simulink model "UZ_EnDat_be4_adding_bidirectional_clk_shift"  (R2024a)
settings: Solver=FixedStepDiscrete  StartTime=0  StopTime=0.02  FixedStep=1.0E-8  RelTol=1e-3
model workspace (MAT data in the model file):
  Select = 0
libraries: hdlsllib x776, simulink x28, simulink_extras x3
(part 4 of 9)

== system UZ_EnDat_be4_adding_bidirectional_clk_shift/UZ_ENDAT/ManualSerializeWrap/ManualSerializer ==
  CLK : Inport
  SLOWCLCK : Inport  Port=2
  DATA : Inport  Port=3
  reset : Inport  Port=4
  Constant3 : Constant  Value=0  OutDataTypeStr=boolean  SampleTime=-1
  Delay1 : Delay  DelayLength=1
  Multiport Switch : MultiPortSwitch  Inputs=6  DataPortForDefault=Additional data port  DiagnosticForDefault=None  SaturateOnIntegerOverflow=off  InputSameDT=off
  Terminator{1..10} (10 alike) : Terminator
  WORDTOBOOL : Subsystem  TreatAsAtomicUnit=on
  ramwatcher : Subsystem  TreatAsAtomicUnit=on
      settings: LibrarySourceBlock=|
      | hdlsllib/Ports &
      | Subsystems/Triggered
      | Subsystem
  valin : Outport
  wires:
  SLOWCLCK/1 -> ramwatcher/Trigger
  DATA/1 -> WORDTOBOOL/1(DATAIN)
  Multiport Switch/1 -> valin/1
  CLK/1 -> WORDTOBOOL/Trigger
  Delay1/1 -> ramwatcher/1(In1)
  Constant3/1 -> Multiport Switch/8
  reset/1 -> ramwatcher/2(reset)
  WORDTOBOOL/1(DATAOUT0) -> Multiport Switch/7
  WORDTOBOOL/2(DATAOUT1) -> Multiport Switch/6
  WORDTOBOOL/3(DATAOUT2) -> Multiport Switch/5
  WORDTOBOOL/4(DATAOUT3) -> Multiport Switch/4
  WORDTOBOOL/5(DATAOUT4) -> Multiport Switch/3
  WORDTOBOOL/6(DATAOUT5) -> Multiport Switch/2
  WORDTOBOOL/9(DATAOUT8) -> Terminator2/1
  WORDTOBOOL/10(DATAOUT9) -> Terminator3/1
  WORDTOBOOL/11(DATAOUT10) -> Terminator4/1
  WORDTOBOOL/12(DATAOUT11) -> Terminator5/1
  WORDTOBOOL/13(DATAOUT12) -> Terminator6/1
  WORDTOBOOL/14(DATAOUT13) -> Terminator7/1
  WORDTOBOOL/15(DATAOUT14) -> Terminator8/1
  WORDTOBOOL/16(DATAOUT15) -> Terminator9/1
  WORDTOBOOL/7(DATAOUT6) -> Terminator1/1
  WORDTOBOOL/8(DATAOUT7) -> Terminator10/1
  ramwatcher/1(SEL) -> Multiport Switch/1, Delay1/1

== system UZ_EnDat_be4_adding_bidirectional_clk_shift/UZ_ENDAT/RESPONSESLICER3X/19BITSLICER ==
  DATA : Inport
  DATA1 : Inport  Port=2
  DATA2 : Inport  Port=3
  Enable : EnablePort
  Terminator : Terminator
  Terminator1 : Terminator
  responseslicer : Subsystem
      settings: LibrarySourceBlock=|
      | hdlsllib/Ports &
      | Subsystems/Subsystem
  responseslicer1 : Subsystem
      settings: LibrarySourceBlock=|
      | hdlsllib/Ports &
      | Subsystems/Subsystem
  responseslicer2 : Subsystem
      settings: LibrarySourceBlock=|
      | hdlsllib/Ports &
      | Subsystems/Subsystem
  CRC : Outport  InitialOutput=0
  payload : Outport  Port=2  InitialOutput=0
  CRC1 : Outport  Port=3  InitialOutput=0
  payload1 : Outport  Port=4  InitialOutput=0
  CRC2 : Outport  Port=5  InitialOutput=0
  payload2 : Outport  Port=6  InitialOutput=0
  sensorerror : Outport  Port=7  InitialOutput=0
  wires:
  DATA1/1 -> responseslicer1/1(DATA)
  DATA/1 -> responseslicer/1(DATA)
  responseslicer/2(payload) -> payload/1
  responseslicer1/2(payload) -> payload1/1
  responseslicer2/2(payload) -> payload2/1
  responseslicer/1(CRC) -> CRC/1
  DATA2/1 -> responseslicer2/1(DATA)
  responseslicer1/1(CRC) -> CRC1/1
  responseslicer2/1(CRC) -> CRC2/1
  responseslicer/3(error) -> sensorerror/1
  responseslicer1/3(error) -> Terminator/1
  responseslicer2/3(error) -> Terminator1/1

== system UZ_EnDat_be4_adding_bidirectional_clk_shift/UZ_ENDAT/RESPONSESLICER3X/21BITSLICER ==
  DATA : Inport
  DATA1 : Inport  Port=2
  DATA2 : Inport  Port=3
  Enable : EnablePort
  Terminator : Terminator
  Terminator1 : Terminator
  responseslicer : Subsystem
      settings: LibrarySourceBlock=|
      | hdlsllib/Ports &
      | Subsystems/Subsystem
  responseslicer3 : Subsystem
      settings: LibrarySourceBlock=|
      | hdlsllib/Ports &
      | Subsystems/Subsystem
  responseslicer4 : Subsystem
      settings: LibrarySourceBlock=|
      | hdlsllib/Ports &
      | Subsystems/Subsystem
  CRC : Outport  InitialOutput=0
  payload : Outport  Port=2  InitialOutput=0
  CRC1 : Outport  Port=3  InitialOutput=0
  payload1 : Outport  Port=4  InitialOutput=0
  CRC2 : Outport  Port=5  InitialOutput=0
  payload2 : Outport  Port=6  InitialOutput=0
  sensorerror : Outport  Port=7  InitialOutput=0
  wires:
  DATA1/1 -> responseslicer4/1(DATA)
  DATA/1 -> responseslicer/1(DATA)
  responseslicer/2(payload) -> payload/1
  responseslicer4/2(payload) -> payload1/1
  responseslicer3/2(payload) -> payload2/1
  responseslicer/1(CRC) -> CRC/1
  DATA2/1 -> responseslicer3/1(DATA)
  responseslicer4/1(CRC) -> CRC1/1
  responseslicer3/1(CRC) -> CRC2/1
  responseslicer/3(error) -> sensorerror/1
  responseslicer4/3(error) -> Terminator/1
  responseslicer3/3(error) -> Terminator1/1

== system UZ_EnDat_be4_adding_bidirectional_clk_shift/UZ_ENDAT/RESPONSESLICER3X/23BITSLICER ==
  DATA : Inport
  DATA1 : Inport  Port=2
  DATA2 : Inport  Port=3
  Enable : EnablePort
  Terminator : Terminator
  Terminator1 : Terminator
  responseslicer : Subsystem
      settings: LibrarySourceBlock=|
      | hdlsllib/Ports &
      | Subsystems/Subsystem
  responseslicer1 : Subsystem
      settings: LibrarySourceBlock=|
      | hdlsllib/Ports &
      | Subsystems/Subsystem
  responseslicer2 : Subsystem
      settings: LibrarySourceBlock=|
      | hdlsllib/Ports &
      | Subsystems/Subsystem
  CRC : Outport  InitialOutput=0
  payload : Outport  Port=2  InitialOutput=0
  CRC1 : Outport  Port=3  InitialOutput=0
  payload1 : Outport  Port=4  InitialOutput=0
  CRC2 : Outport  Port=5  InitialOutput=0
  payload2 : Outport  Port=6  InitialOutput=0
  sensorerror : Outport  Port=7  InitialOutput=0
  wires:
  DATA1/1 -> responseslicer1/1(DATA)
  DATA/1 -> responseslicer/1(DATA)
  responseslicer/2(payload) -> payload/1
  responseslicer1/2(payload) -> payload1/1
  responseslicer2/2(payload) -> payload2/1
  responseslicer/1(CRC) -> CRC/1
  DATA2/1 -> responseslicer2/1(DATA)
  responseslicer1/1(CRC) -> CRC1/1
  responseslicer2/1(CRC) -> CRC2/1
  responseslicer/3(error) -> sensorerror/1
  responseslicer1/3(error) -> Terminator/1
  responseslicer2/3(error) -> Terminator1/1

== system UZ_EnDat_be4_adding_bidirectional_clk_shift/UZ_ENDAT/RESPONSESLICER3X/25BITSLICER ==
  DATA : Inport
  DATA1 : Inport  Port=2
  DATA2 : Inport  Port=3
  Enable : EnablePort
  Terminator : Terminator
  Terminator1 : Terminator
  responseslicer : Subsystem
      settings: LibrarySourceBlock=|
      | hdlsllib/Ports &
      | Subsystems/Subsystem
  responseslicer1 : Subsystem
      settings: LibrarySourceBlock=|
      | hdlsllib/Ports &
      | Subsystems/Subsystem
  responseslicer2 : Subsystem
      settings: LibrarySourceBlock=|
      | hdlsllib/Ports &
      | Subsystems/Subsystem
  CRC : Outport  InitialOutput=0
  payload : Outport  Port=2  InitialOutput=0
  CRC1 : Outport  Port=3  InitialOutput=0
  payload1 : Outport  Port=4  InitialOutput=0
  CRC2 : Outport  Port=5  InitialOutput=0
  payload2 : Outport  Port=6  InitialOutput=0
  sensorerror : Outport  Port=7  InitialOutput=0
  wires:
  DATA1/1 -> responseslicer1/1(DATA)
  DATA/1 -> responseslicer/1(DATA)
  responseslicer/2(payload) -> payload/1
  responseslicer1/2(payload) -> payload1/1
  responseslicer2/2(payload) -> payload2/1
  responseslicer/1(CRC) -> CRC/1
  DATA2/1 -> responseslicer2/1(DATA)
  responseslicer1/1(CRC) -> CRC1/1
  responseslicer2/1(CRC) -> CRC2/1
  responseslicer/3(error) -> sensorerror/1
  responseslicer1/3(error) -> Terminator/1
  responseslicer2/3(error) -> Terminator1/1

== system UZ_EnDat_be4_adding_bidirectional_clk_shift/UZ_ENDAT/RESPONSESLICER3X/27BITSLICER ==
  DATA : Inport
  DATA1 : Inport  Port=2
  DATA2 : Inport  Port=3
  Enable : EnablePort
  Terminator : Terminator
  Terminator1 : Terminator
  responseslicer : Subsystem
      settings: LibrarySourceBlock=|
      | hdlsllib/Ports &
      | Subsystems/Subsystem
  responseslicer1 : Subsystem
      settings: LibrarySourceBlock=|
      | hdlsllib/Ports &
      | Subsystems/Subsystem
  responseslicer2 : Subsystem
      settings: LibrarySourceBlock=|
      | hdlsllib/Ports &
      | Subsystems/Subsystem
  CRC : Outport  InitialOutput=0
  payload : Outport  Port=2  InitialOutput=0
  CRC1 : Outport  Port=3  InitialOutput=0
  payload1 : Outport  Port=4  InitialOutput=0
  CRC2 : Outport  Port=5  InitialOutput=0
  payload2 : Outport  Port=6  InitialOutput=0
  sensorerror : Outport  Port=7  InitialOutput=0
  wires:
  DATA1/1 -> responseslicer1/1(DATA)
  DATA/1 -> responseslicer/1(DATA)
  responseslicer/2(payload) -> payload/1
  responseslicer1/2(payload) -> payload1/1
  responseslicer2/2(payload) -> payload2/1
  responseslicer/1(CRC) -> CRC/1
  DATA2/1 -> responseslicer2/1(DATA)
  responseslicer1/1(CRC) -> CRC1/1
  responseslicer2/1(CRC) -> CRC2/1
  responseslicer/3(error) -> sensorerror/1
  responseslicer1/3(error) -> Terminator/1
  responseslicer2/3(error) -> Terminator1/1

== system UZ_EnDat_be4_adding_bidirectional_clk_shift/UZ_ENDAT/timingprovider/Subsystem1 ==
  Trigger : TriggerPort  VariantControl=(inherit)  PortDimensions=1
  HDL Counter : hdlsllib/Sources/HDL Counter  CountType=Count limited  CountInit=0  CountStep=1  CountMax=3  CountFromType=Initial value  CountFrom=0  CountResetPort=off  CountLoadPort=off  CountEnbPort=off  CountDirPort=off  CountHitOutputPort=on  CountDataType=Unsigned  CountWordLen=2  CountFracLen=0  CountSampTime=-1
  valin1 : Outport  InitialOutput=0
  valin2 : Outport  Port=2  InitialOutput=0
  wires:
  HDL Counter/1 -> valin1/1
  HDL Counter/2 -> valin2/1

== system UZ_EnDat_be4_adding_bidirectional_clk_shift/UZ_ENDAT/timingprovider/Subsystem2 ==
  elapsed : Inport
  clkcnt : Inport  Port=2
  Compare To Constant1 : hdlsllib/Logic and Bit Operations/Compare To Constant  relop===  const=3  OutDataTypeStr=boolean
  Delay1 : Delay  DelayLength=1
  Detect Increase : simulink/Logic and Bit Operations/Detect Increase  vinit=0  OutDataTypeStr=boolean
      settings: LibrarySourceBlock=|
      | hdlsllib/Logic and Bit
      | Operations/Detect
      | Increase
  Gain : Gain  Gain=10  ParamMin=10  ParamMax=10  ParamDataTypeStr=uint8  OutDataTypeStr=uint32  RndMeth=Simplest
  Switch : Switch  Criteria=u2 > Threshold  SaturateOnIntegerOverflow=off  InputSameDT=off
  ns elapsed : Outport
  wires:
  Detect Increase/1 -> Switch/2
  clkcnt/1 -> Switch/1
  Switch/1 -> Gain/1, Delay1/1
  Delay1/1 -> Switch/3
  elapsed/1 -> Compare To Constant1/1
  Gain/1 -> ns elapsed/1  "ns elapsed"
  Compare To Constant1/1 -> Detect Increase/1

== system UZ_EnDat_be4_adding_bidirectional_clk_shift/UZ_ENDAT/timingprovider/Subsystem3 ==
  elapsed : Inport
  clkcnt : Inport  Port=2
  Compare To Constant1 : hdlsllib/Logic and Bit Operations/Compare To Constant  relop===  const=3  OutDataTypeStr=boolean
  Constant : Constant  Value=10  OutDataTypeStr=uint8  SampleTime=-1
  Delay1 : Delay  DelayLength=1
  Detect Increase : simulink/Logic and Bit Operations/Detect Increase  vinit=0  OutDataTypeStr=boolean
      settings: LibrarySourceBlock=|
      | hdlsllib/Logic and Bit
      | Operations/Detect
      | Increase
  Switch : Switch  Criteria=u2 > Threshold  SaturateOnIntegerOverflow=off  InputSameDT=off
  nsproduct : Product  OutDataTypeStr=uint32  RndMeth=Simplest
  ns elapsed : Outport
  wires:
  Detect Increase/1 -> Switch/2
  clkcnt/1 -> Switch/1
  Switch/1 -> nsproduct/2, Delay1/1
  Delay1/1 -> Switch/3
  elapsed/1 -> Compare To Constant1/1
  nsproduct/1 -> ns elapsed/1  "ns elapsed"
  Constant/1 -> nsproduct/1
  Compare To Constant1/1 -> Detect Increase/1

== system UZ_EnDat_be4_adding_bidirectional_clk_shift/UZ_ENDAT/timingprovider/Subsystem4 ==
  reset : Inport
  Trigger : TriggerPort  TriggerType=either  VariantControl=(inherit)  PortDimensions=1
  Delay : Delay  Commented=through  DelayLength=1
  HDL Counter : hdlsllib/Sources/HDL Counter  CountType=Count limited  CountInit=0  CountStep=1  CountMax=65535  CountFromType=Initial value  CountFrom=0  CountResetPort=on  CountLoadPort=off  CountEnbPort=off  CountDirPort=off  CountHitOutputPort=off  CountDataType=Unsigned  CountWordLen=16  CountFracLen=0  CountSampTime=1
  Scope : Scope
  valin1 : Outport  InitialOutput=0
  wires:
  reset/1 -> Delay/1
  HDL Counter/1 -> valin1/1, Scope/1
  Delay/1 -> HDL Counter/1

== system UZ_EnDat_be4_adding_bidirectional_clk_shift/UZ_ENDAT/timingprovider/Subsystem5 ==
  elapsed : Inport
  clkcnt : Inport  Port=2
  Compare To Constant1 : hdlsllib/Logic and Bit Operations/Compare To Constant  relop===  const=2  OutDataTypeStr=boolean
  Delay1 : Delay  DelayLength=1
  Detect Increase : simulink/Logic and Bit Operations/Detect Increase  vinit=0  OutDataTypeStr=boolean
      settings: LibrarySourceBlock=|
      | hdlsllib/Logic and Bit
      | Operations/Detect
      | Increase
  Gain : Gain  Gain=10  ParamMin=10  ParamMax=10  ParamDataTypeStr=uint8  OutDataTypeStr=uint32  RndMeth=Simplest
  Switch : Switch  Criteria=u2 > Threshold  SaturateOnIntegerOverflow=off  InputSameDT=off
  ns elapsed : Outport
  wires:
  Detect Increase/1 -> Switch/2
  clkcnt/1 -> Switch/1
  Switch/1 -> Gain/1, Delay1/1
  Delay1/1 -> Switch/3
  elapsed/1 -> Compare To Constant1/1
  Gain/1 -> ns elapsed/1  "ns elapsed"
  Compare To Constant1/1 -> Detect Increase/1

== system UZ_EnDat_be4_adding_bidirectional_clk_shift/UZ_ENDAT/timingprovider/Subsystem6 ==
  elapsed : Inport
  clkcnt : Inport  Port=2
  Compare To Constant1 : hdlsllib/Logic and Bit Operations/Compare To Constant  relop===  const=3  OutDataTypeStr=boolean
  Constant : Constant  Value=10  OutDataTypeStr=uint8  SampleTime=-1
  Delay1 : Delay  DelayLength=1
  Detect Increase : simulink/Logic and Bit Operations/Detect Increase  vinit=0  OutDataTypeStr=boolean
      settings: LibrarySourceBlock=|
      | hdlsllib/Logic and Bit
      | Operations/Detect
      | Increase
  Switch : Switch  Criteria=u2 > Threshold  SaturateOnIntegerOverflow=off  InputSameDT=off
  nsproduct : Product  OutDataTypeStr=uint32  RndMeth=Simplest
  ns elapsed : Outport
  wires:
  Detect Increase/1 -> Switch/2
  clkcnt/1 -> Switch/1
  Switch/1 -> nsproduct/2, Delay1/1
  Delay1/1 -> Switch/3
  elapsed/1 -> Compare To Constant1/1
  nsproduct/1 -> ns elapsed/1  "ns elapsed"
  Constant/1 -> nsproduct/1
  Compare To Constant1/1 -> Detect Increase/1

== system UZ_EnDat_be4_adding_bidirectional_clk_shift/UZ_ENDAT/timingprovider/Subsystem7 ==
  elapsed : Inport
  clkcnt : Inport  Port=2
  Compare To Constant1 : hdlsllib/Logic and Bit Operations/Compare To Constant  relop===  const=2  OutDataTypeStr=boolean
  Constant : Constant  Value=10  OutDataTypeStr=uint8  SampleTime=-1
  Delay1 : Delay  DelayLength=1
  Detect Increase : simulink/Logic and Bit Operations/Detect Increase  vinit=0  OutDataTypeStr=boolean
      settings: LibrarySourceBlock=|
      | hdlsllib/Logic and Bit
      | Operations/Detect
      | Increase
  Switch : Switch  Criteria=u2 > Threshold  SaturateOnIntegerOverflow=off  InputSameDT=off
  nsproduct : Product  OutDataTypeStr=uint32  RndMeth=Simplest
  ns elapsed : Outport
  wires:
  Detect Increase/1 -> Switch/2
  clkcnt/1 -> Switch/1
  Switch/1 -> nsproduct/2, Delay1/1
  Delay1/1 -> Switch/3
  elapsed/1 -> Compare To Constant1/1
  nsproduct/1 -> ns elapsed/1  "ns elapsed"
  Constant/1 -> nsproduct/1
  Compare To Constant1/1 -> Detect Increase/1

== system UZ_EnDat_be4_adding_bidirectional_clk_shift/UZ_ENDAT/timingprovideralternative/Subsystem1 ==
  Trigger : TriggerPort  VariantControl=(inherit)  PortDimensions=1
  HDL Counter : hdlsllib/Sources/HDL Counter  CountType=Count limited  CountInit=0  CountStep=1  CountMax=3  CountFromType=Initial value  CountFrom=0  CountResetPort=off  CountLoadPort=off  CountEnbPort=off  CountDirPort=off  CountHitOutputPort=on  CountDataType=Unsigned  CountWordLen=2  CountFracLen=0  CountSampTime=-1
  valin1 : Outport  InitialOutput=0
  valin2 : Outport  Port=2  InitialOutput=0
  wires:
  HDL Counter/1 -> valin1/1
  HDL Counter/2 -> valin2/1

== system UZ_EnDat_be4_adding_bidirectional_clk_shift/UZ_ENDAT/timingprovideralternative/Subsystem2 ==
  elapsed : Inport
  clkcnt : Inport  Port=2
  Compare To Constant1 : hdlsllib/Logic and Bit Operations/Compare To Constant  relop===  const=3  OutDataTypeStr=boolean
  Constant : Constant  Value=10  OutDataTypeStr=uint32  SampleTime=-1
  Delay1 : Delay  DelayLength=1
  Detect Increase : simulink/Logic and Bit Operations/Detect Increase  vinit=0  OutDataTypeStr=boolean
      settings: LibrarySourceBlock=|
      | hdlsllib/Logic and Bit
      | Operations/Detect
      | Increase
  Switch : Switch  Criteria=u2 > Threshold  SaturateOnIntegerOverflow=off  InputSameDT=off
  nsproduct : Product  OutDataTypeStr=uint32  RndMeth=Simplest  SaturateOnIntegerOverflow=on
  ns elapsed : Outport
  wires:
  Detect Increase/1 -> Switch/2
  clkcnt/1 -> Switch/1
  Switch/1 -> nsproduct/2, Delay1/1
  Delay1/1 -> Switch/3
  elapsed/1 -> Compare To Constant1/1
  nsproduct/1 -> ns elapsed/1  "ns elapsed"
  Constant/1 -> nsproduct/1
  Compare To Constant1/1 -> Detect Increase/1

== system UZ_EnDat_be4_adding_bidirectional_clk_shift/UZ_ENDAT/timingprovideralternative/Subsystem3 ==
  elapsed : Inport
  clkcnt : Inport  Port=2
  Compare To Constant1 : hdlsllib/Logic and Bit Operations/Compare To Constant  relop===  const=2  OutDataTypeStr=boolean
  Constant : Constant  Value=10  OutDataTypeStr=uint32  SampleTime=-1
  Delay1 : Delay  DelayLength=1
  Detect Increase : simulink/Logic and Bit Operations/Detect Increase  vinit=0  OutDataTypeStr=boolean
      settings: LibrarySourceBlock=|
      | hdlsllib/Logic and Bit
      | Operations/Detect
      | Increase
  Switch : Switch  Criteria=u2 > Threshold  SaturateOnIntegerOverflow=off  InputSameDT=off
  nsproduct : Product  OutDataTypeStr=uint32  RndMeth=Simplest  SaturateOnIntegerOverflow=on
  ns elapsed : Outport
  wires:
  Detect Increase/1 -> Switch/2
  clkcnt/1 -> Switch/1
  Switch/1 -> nsproduct/2, Delay1/1
  Delay1/1 -> Switch/3
  elapsed/1 -> Compare To Constant1/1
  nsproduct/1 -> ns elapsed/1  "ns elapsed"
  Constant/1 -> nsproduct/1
  Compare To Constant1/1 -> Detect Increase/1

== system UZ_EnDat_be4_adding_bidirectional_clk_shift/UZ_ENDAT/timingprovideralternative/Subsystem4 ==
  reset : Inport
  Delay : Delay  Commented=through  DelayLength=1
  HDL Counter : hdlsllib/Sources/HDL Counter  CountType=Count limited  CountInit=0  CountStep=1  CountMax=214748364  CountFromType=Initial value  CountFrom=0  CountResetPort=on  CountLoadPort=off  CountEnbPort=off  CountDirPort=off  CountHitOutputPort=off  CountDataType=Unsigned  CountWordLen=32  CountFracLen=0  CountSampTime=1
  Scope : Scope
  valin1 : Outport  InitialOutput=0
  wires:
  reset/1 -> Delay/1
  HDL Counter/1 -> valin1/1, Scope/1
  Delay/1 -> HDL Counter/1

== system UZ_EnDat_be4_adding_bidirectional_clk_shift/UZ_ENDAT/timingprovideralternative/timingproviderold ==
  wrok : Inport  OutDataTypeStr=boolean
  clk : Inport  Port=2  OutDataTypeStr=boolean
  Compare To Constant1 : hdlsllib/Logic and Bit Operations/Compare To Constant  relop===  const=0  OutDataTypeStr=boolean
  Constant3 : Constant  Commented=on  Value=0x7FFFF0  OutDataTypeStr=uint32  SampleTime=-1
  Constant4 : Constant  Commented=on  Value=0x7FFFFF  OutDataTypeStr=uint32  SampleTime=-1
  Logical Operator : Logic  Operator=OR  AllPortsSameDT=off  OutDataTypeStr=boolean
  Subsystem1 : Subsystem
  Subsystem2 : Subsystem
  Subsystem3 : Subsystem
  Subsystem4 : Subsystem
  timeelapsed2cycl : Outport  OutDataTypeStr=uint32
  timeelapsed1cycl : Outport  Port=2  OutDataTypeStr=uint32
  wires:
  wrok/1 -> Subsystem1/Trigger
  Subsystem2/1(ns elapsed) -> timeelapsed2cycl/1
  Subsystem3/1(ns elapsed) -> timeelapsed1cycl/1
  Subsystem1/1(valin1) -> Compare To Constant1/1, Subsystem3/1(elapsed), Subsystem2/1(elapsed)
  Logical Operator/1 -> Subsystem4/1(reset)
  Compare To Constant1/1 -> Logical Operator/2
  clk/1 -> Subsystem4/Trigger
  Subsystem4/1(valin1) -> Subsystem2/2(clkcnt), Subsystem3/2(clkcnt)
  Subsystem1/2(valin2) -> Logical Operator/1

== system UZ_EnDat_be4_adding_bidirectional_clk_shift/UZ_ENDAT/timingproviderold1/Subsystem1 ==
  Trigger : TriggerPort  VariantControl=(inherit)  PortDimensions=1
  HDL Counter : hdlsllib/Sources/HDL Counter  CountType=Count limited  CountInit=0  CountStep=1  CountMax=3  CountFromType=Initial value  CountFrom=0  CountResetPort=off  CountLoadPort=off  CountEnbPort=off  CountDirPort=off  CountHitOutputPort=on  CountDataType=Unsigned  CountWordLen=2  CountFracLen=0  CountSampTime=-1
  valin1 : Outport  InitialOutput=0
  valin2 : Outport  Port=2  InitialOutput=0
  wires:
  HDL Counter/1 -> valin1/1
  HDL Counter/2 -> valin2/1

== system UZ_EnDat_be4_adding_bidirectional_clk_shift/UZ_ENDAT/timingproviderold1/Subsystem2 ==
  elapsed : Inport
  clkcnt : Inport  Port=2
  Compare To Constant1 : hdlsllib/Logic and Bit Operations/Compare To Constant  relop===  const=3  OutDataTypeStr=boolean
  Constant : Constant  Value=20  OutDataTypeStr=uint32  SampleTime=-1
  Delay1 : Delay  DelayLength=1
  Detect Increase : simulink/Logic and Bit Operations/Detect Increase  vinit=0  OutDataTypeStr=boolean
      settings: LibrarySourceBlock=|
      | hdlsllib/Logic and Bit
      | Operations/Detect
      | Increase
  Switch : Switch  Criteria=u2 > Threshold  SaturateOnIntegerOverflow=off  InputSameDT=off
  nsproduct : Product  OutDataTypeStr=uint32  RndMeth=Simplest  SaturateOnIntegerOverflow=on
  ns elapsed : Outport
  wires:
  Detect Increase/1 -> Switch/2
  clkcnt/1 -> Switch/1
  Switch/1 -> nsproduct/2, Delay1/1
  Delay1/1 -> Switch/3
  elapsed/1 -> Compare To Constant1/1
  nsproduct/1 -> ns elapsed/1  "ns elapsed"
  Constant/1 -> nsproduct/1
  Compare To Constant1/1 -> Detect Increase/1

== system UZ_EnDat_be4_adding_bidirectional_clk_shift/UZ_ENDAT/timingproviderold1/Subsystem3 ==
  elapsed : Inport
  clkcnt : Inport  Port=2
  Compare To Constant1 : hdlsllib/Logic and Bit Operations/Compare To Constant  relop===  const=2  OutDataTypeStr=boolean
  Constant : Constant  Value=20  OutDataTypeStr=uint32  SampleTime=-1
  Delay1 : Delay  DelayLength=1
  Detect Increase : simulink/Logic and Bit Operations/Detect Increase  vinit=0  OutDataTypeStr=boolean
      settings: LibrarySourceBlock=|
      | hdlsllib/Logic and Bit
      | Operations/Detect
      | Increase
  Switch : Switch  Criteria=u2 > Threshold  SaturateOnIntegerOverflow=off  InputSameDT=off
  nsproduct : Product  OutDataTypeStr=uint32  RndMeth=Simplest  SaturateOnIntegerOverflow=on
  ns elapsed : Outport
  wires:
  Detect Increase/1 -> Switch/2
  clkcnt/1 -> Switch/1
  Switch/1 -> nsproduct/2, Delay1/1
  Delay1/1 -> Switch/3
  elapsed/1 -> Compare To Constant1/1
  nsproduct/1 -> ns elapsed/1  "ns elapsed"
  Constant/1 -> nsproduct/1
  Compare To Constant1/1 -> Detect Increase/1

== system UZ_EnDat_be4_adding_bidirectional_clk_shift/UZ_ENDAT/timingproviderold1/Subsystem4 ==
  reset : Inport
  Trigger : TriggerPort  VariantControl=(inherit)  PortDimensions=1
  Delay : Delay  Commented=through  DelayLength=1
  HDL Counter : hdlsllib/Sources/HDL Counter  CountType=Count limited  CountInit=0  CountStep=1  CountMax=214748364  CountFromType=Initial value  CountFrom=0  CountResetPort=on  CountLoadPort=off  CountEnbPort=off  CountDirPort=off  CountHitOutputPort=off  CountDataType=Unsigned  CountWordLen=32  CountFracLen=0  CountSampTime=1
  Scope : Scope
  valin1 : Outport  InitialOutput=0
  wires:
  reset/1 -> Delay/1
  HDL Counter/1 -> valin1/1, Scope/1
  Delay/1 -> HDL Counter/1

== system UZ_EnDat_be4_adding_bidirectional_clk_shift/UZ_ENDAT_ABZ_ADDON/ManualSerialize1/FF1 ==
  SET : Inport
  RST : Inport  Port=2
  S-R Flip-Flop : simulink_extras/Flip Flops/S-R Flip-Flop  initial_condition=0
  OQ : Outport
  NOQ : Outport  Port=2
  wires:
  SET/1 -> S-R Flip-Flop/1
  RST/1 -> S-R Flip-Flop/2
  S-R Flip-Flop/1 -> OQ/1
  S-R Flip-Flop/2 -> NOQ/1

== system UZ_EnDat_be4_adding_bidirectional_clk_shift/UZ_ENDAT_ABZ_ADDON/ManualSerialize1/SetZero64modified ==
  valin : Inport
  setzero : Inport  Port=2  OutDataTypeStr=boolean
  Trigger : TriggerPort  TriggerType=either  VariantControl=(inherit)
  Constant2 : Constant  Value=0  OutDataTypeStr=uint64  SampleTime=-1
  Index Vector1 : MultiPortSwitch  DataPortOrder=Zero-based contiguous  Inputs=2  zeroidx=on  OutDataTypeStr=uint64  SaturateOnIntegerOverflow=off  InputSameDT=off
  valueout : Outport  InitialOutput=1  VectorParamsAs1DForOutWhenUnconnected=off
  wires:
  valin/1 -> Index Vector1/2
  Index Vector1/1 -> valueout/1
  Constant2/1 -> Index Vector1/3
  setzero/1 -> Index Vector1/1

== system UZ_EnDat_be4_adding_bidirectional_clk_shift/UZ_ENDAT_ABZ_ADDON/ManualSerialize1/Storage1 ==
  Data : Inport
  Write : Inport  Port=2  OutDataTypeStr=boolean
  Compare To Zero : hdlsllib/Logic and Bit Operations/Compare To Zero  relop===  OutDataTypeStr=boolean
  Delay2 : Delay  DelayLength=1
  Logical Operator1 : Logic  AllPortsSameDT=off  OutDataTypeStr=boolean
  Logical Operator2 : Logic  Operator=NOT  AllPortsSameDT=off  OutDataTypeStr=boolean
  Single Port RAM System : hdlsllib/HDL RAMs/Single Port RAM System  Commented=on  RAMType=Single port  AsyncRead=off  WriteOutputValue=Old data  RAMInitialValue=0  allowBusInputs=off  WritesHaveOutput=on  NumReads=0  NumWrites=1  SimulateUsing=Code generation
  Switch : Switch  Criteria=u2 > Threshold  SaturateOnIntegerOverflow=off  InputSameDT=off
  prolonger : Subsystem  Commented=through
  out : Outport
  wrok : Outport  Port=2  OutDataTypeStr=boolean
  wires:
  Switch/1 -> Delay2/1
  Compare To Zero/1 -> Logical Operator2/1
  Logical Operator2/1 -> Logical Operator1/2
  prolonger/1(out) -> wrok/1
  Data/1 -> Compare To Zero/1, Switch/1
  Delay2/1 -> out/1, Switch/3
  Logical Operator1/1 -> prolonger/1(in), Switch/2
  Write/1 -> Logical Operator1/1

== system UZ_EnDat_be4_adding_bidirectional_clk_shift/UZ_ENDAT_ABZ_ADDON/ManualSerialize1/Storage16 ==
  Data : Inport
  Write : Inport  Port=2  OutDataTypeStr=boolean
  Compare To Zero : hdlsllib/Logic and Bit Operations/Compare To Zero  relop===  OutDataTypeStr=boolean
  Logical Operator : Logic  Operator=NOT  AllPortsSameDT=off  OutDataTypeStr=boolean
  Logical Operator1 : Logic  Inputs=3  AllPortsSameDT=off  OutDataTypeStr=boolean
  Logical Operator2 : Logic  Operator=NOT  AllPortsSameDT=off  OutDataTypeStr=boolean
  Logical Operator3 : Logic  Inputs=3  AllPortsSameDT=off  OutDataTypeStr=boolean
  Logical Operator4 : Logic  Operator=NOT  AllPortsSameDT=off  OutDataTypeStr=boolean
  Relational Operator : RelationalOperator  Operator===  OutDataTypeStr=boolean  InputSameDT=off
  Scope : Scope  NumInputPorts=5
  Single Port RAM System : hdlsllib/HDL RAMs/Single Port RAM System  RAMType=Single port  AsyncRead=off  WriteOutputValue=Old data  RAMInitialValue=0  allowBusInputs=off  WritesHaveOutput=on  NumReads=0  NumWrites=1  SimulateUsing=Code generation
  adress : Constant  Value=6  OutDataTypeStr=uint8  SampleTime=-1
  out : Outport
  wrok : Outport  Port=2  OutDataTypeStr=boolean
  wires:
  Single Port RAM System/1 -> Relational Operator/1, out/1
  Data/1 -> Compare To Zero/1, Single Port RAM System/1, Relational Operator/2
  adress/1 -> Single Port RAM System/2
  Relational Operator/1 -> Scope/1, Logical Operator/1, Logical Operator3/1
  Logical Operator/1 -> Logical Operator1/2
  Write/1 -> Scope/4, Logical Operator4/1, Logical Operator1/1
  Compare To Zero/1 -> Logical Operator2/1
  Logical Operator1/1 -> Single Port RAM System/3, Scope/5
  Logical Operator3/1 -> wrok/1, Scope/2
  Logical Operator4/1 -> Logical Operator3/3
  Logical Operator2/1 -> Logical Operator1/3, Logical Operator3/2, Scope/3

== system UZ_EnDat_be4_adding_bidirectional_clk_shift/UZ_ENDAT_ABZ_ADDON/ManualSerialize1/Storage2 ==
  Data : Inport
  Write : Inport  Port=2  OutDataTypeStr=boolean
  Compare To Zero : hdlsllib/Logic and Bit Operations/Compare To Zero  relop===  OutDataTypeStr=boolean
  Delay : Delay  DelayLength=1
  Delay2 : Delay  DelayLength=1
  Logical Operator1 : Logic  AllPortsSameDT=off  OutDataTypeStr=boolean
  Logical Operator2 : Logic  Operator=NOT  AllPortsSameDT=off  OutDataTypeStr=boolean
  Scope1 : Scope  NumInputPorts=2
  Single Port RAM System : hdlsllib/HDL RAMs/Single Port RAM System  Commented=on  RAMType=Single port  AsyncRead=off  WriteOutputValue=Old data  RAMInitialValue=0  allowBusInputs=off  WritesHaveOutput=on  NumReads=0  NumWrites=1  SimulateUsing=Code generation
  Switch : Switch  Criteria=u2 > Threshold  SaturateOnIntegerOverflow=off  InputSameDT=off
  prolonger : Subsystem
  out : Outport
  wrok : Outport  Port=2  OutDataTypeStr=boolean
  wires:
  Switch/1 -> Delay2/1
  Compare To Zero/1 -> Logical Operator2/1
  Logical Operator1/1 -> Delay/1, Switch/2
  Logical Operator2/1 -> Logical Operator1/2
  prolonger/1(out) -> wrok/1
  Data/1 -> Scope1/1, Compare To Zero/1, Switch/1
  Delay2/1 -> out/1, Switch/3
  Delay/1 -> prolonger/1(in)
  Write/1 -> Logical Operator1/1

== system UZ_EnDat_be4_adding_bidirectional_clk_shift/UZ_ENDAT_ABZ_ADDON/ManualSerialize1/Subsystem ==
  countclk : Inport
  reset : Inport  Port=2
  Delay : Delay  DelayLength=1
  Detect Increase : simulink/Logic and Bit Operations/Detect Increase  vinit=0.0  OutDataTypeStr=boolean
      settings: LibrarySourceBlock=|
      | hdlsllib/Logic and Bit
      | Operations/Detect
      | Increase
  HDL Counter : hdlsllib/Sources/HDL Counter  CountType=Count limited  CountInit=0  CountStep=1  CountMax=51  CountFromType=Initial value  CountFrom=0  CountResetPort=on  CountLoadPort=off  CountEnbPort=on  CountDirPort=off  CountHitOutputPort=off  CountDataType=Unsigned  CountWordLen=8  CountFracLen=0  CountSampTime=1
  Scope : Scope
  valin1 : Outport  InitialOutput=0
  wires:
  countclk/1 -> Detect Increase/1
  Detect Increase/1 -> HDL Counter/2
  reset/1 -> Delay/1
  HDL Counter/1 -> valin1/1, Scope/1
  Delay/1 -> HDL Counter/1

== system UZ_EnDat_be4_adding_bidirectional_clk_shift/UZ_ENDAT_ABZ_ADDON/ManualSerialize1/Triggered Subsystem ==
  DATA : Inport
  valueout : Inport  Port=2
  Trigger : TriggerPort  VariantControl=(inherit)
  Bit Clear : simulink/Logic and Bit Operations/Bit Clear  iBit=50
      settings: LibrarySourceBlock=|
      | hdlsllib/Logic and Bit
      | Operations/Bit Clear
  Bit Set : simulink/Logic and Bit Operations/Bit Set  iBit=50
      settings: LibrarySourceBlock=|
      | hdlsllib/Logic and Bit
      | Operations/Bit Set
  Bit Shift : hdlsllib/Logic and Bit Operations/Bit Shift  mode=Shift Right Logical  N=1
  Display : Display
      settings: Format=binary (Stored Integer)
  Scope : Scope  NumInputPorts=2
  Switch : Switch  Criteria=u2 ~= 0  SaturateOnIntegerOverflow=off  InputSameDT=off
  valin : Outport  InitialOutput=0
  wires:
  DATA/1 -> Scope/1, Switch/2
  valueout/1 -> Bit Clear/1, Bit Set/1, Scope/2
  Bit Set/1 -> Switch/1
  Switch/1 -> Bit Shift/1
  Bit Shift/1 -> Display/1, valin/1
  Bit Clear/1 -> Switch/3

== system UZ_EnDat_be4_adding_bidirectional_clk_shift/UZ_ENDAT_ABZ_ADDON/ManualSerialize1/nibblepadding6 ==
  in : Inport
  padding : Subsystem
  padding1 : Subsystem
  padding2 : Subsystem
  padding3 : Subsystem
  out : Outport
  wires:
  in/1 -> padding3/1(in)
  padding2/1(out) -> padding1/1(in)
  padding3/1(out) -> padding2/1(in)
  padding1/1(out) -> padding/1(in)
  padding/1(out) -> out/1

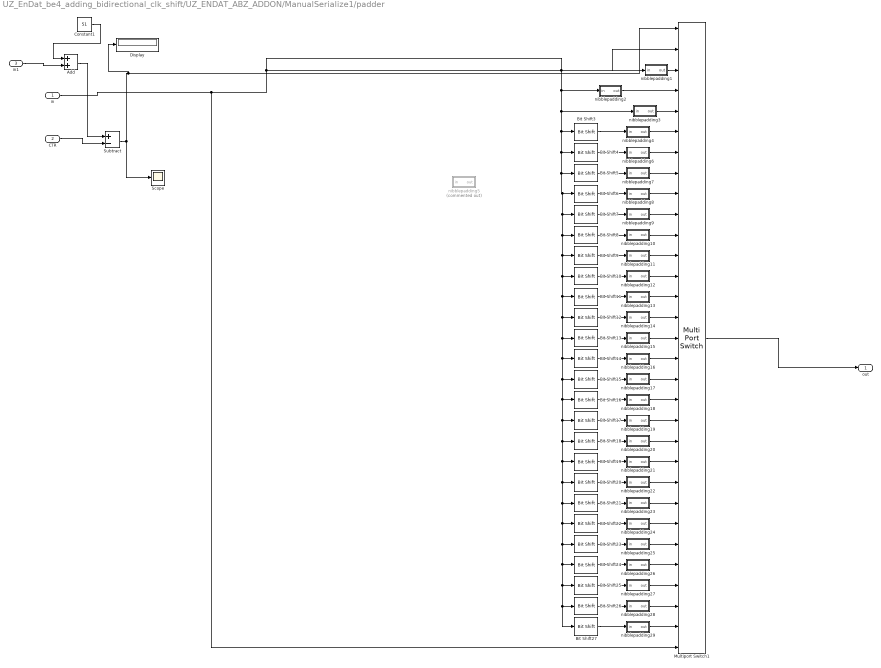
== system UZ_EnDat_be4_adding_bidirectional_clk_shift/UZ_ENDAT_ABZ_ADDON/ManualSerialize1/padder ==
  in : Inport
  CTR : Inport  Port=2
  in1 : Inport  Port=3  OutDataTypeStr=int8
  Add : Sum  OutDataTypeStr=uint8  AccumDataTypeStr=uint8  RndMeth=Simplest
  Bit Shift10 : hdlsllib/Logic and Bit Operations/Bit Shift  mode=Shift Right Logical  N=8
  Bit Shift11 : hdlsllib/Logic and Bit Operations/Bit Shift  mode=Shift Right Logical  N=9
  Bit Shift12 : hdlsllib/Logic and Bit Operations/Bit Shift  mode=Shift Right Logical  N=10
  Bit Shift13 : hdlsllib/Logic and Bit Operations/Bit Shift  mode=Shift Right Logical  N=11
  Bit Shift14 : hdlsllib/Logic and Bit Operations/Bit Shift  mode=Shift Right Logical  N=12
  Bit Shift15 : hdlsllib/Logic and Bit Operations/Bit Shift  mode=Shift Right Logical  N=13
  Bit Shift16 : hdlsllib/Logic and Bit Operations/Bit Shift  mode=Shift Right Logical  N=14
  Bit Shift17 : hdlsllib/Logic and Bit Operations/Bit Shift  mode=Shift Right Logical  N=15
  Bit Shift18 : hdlsllib/Logic and Bit Operations/Bit Shift  mode=Shift Right Logical  N=16
  Bit Shift19 : hdlsllib/Logic and Bit Operations/Bit Shift  mode=Shift Right Logical  N=17
  Bit Shift20 : hdlsllib/Logic and Bit Operations/Bit Shift  mode=Shift Right Logical  N=18
  Bit Shift21 : hdlsllib/Logic and Bit Operations/Bit Shift  mode=Shift Right Logical  N=19
  Bit Shift22 : hdlsllib/Logic and Bit Operations/Bit Shift  mode=Shift Right Logical  N=20
  Bit Shift23 : hdlsllib/Logic and Bit Operations/Bit Shift  mode=Shift Right Logical  N=21
  Bit Shift24 : hdlsllib/Logic and Bit Operations/Bit Shift  mode=Shift Right Logical  N=22
  Bit Shift25 : hdlsllib/Logic and Bit Operations/Bit Shift  mode=Shift Right Logical  N=23
  Bit Shift26 : hdlsllib/Logic and Bit Operations/Bit Shift  mode=Shift Right Logical  N=24
  Bit Shift27 : hdlsllib/Logic and Bit Operations/Bit Shift  mode=Shift Right Logical  N=25
  Bit Shift3 : hdlsllib/Logic and Bit Operations/Bit Shift  mode=Shift Right Logical  N=1
  Bit Shift4 : hdlsllib/Logic and Bit Operations/Bit Shift  mode=Shift Right Logical  N=2
  Bit Shift5 : hdlsllib/Logic and Bit Operations/Bit Shift  mode=Shift Right Logical  N=3
  Bit Shift6 : hdlsllib/Logic and Bit Operations/Bit Shift  mode=Shift Right Logical  N=4
  Bit Shift7 : hdlsllib/Logic and Bit Operations/Bit Shift  mode=Shift Right Logical  N=5
  Bit Shift8 : hdlsllib/Logic and Bit Operations/Bit Shift  mode=Shift Right Logical  N=6
  Bit Shift9 : hdlsllib/Logic and Bit Operations/Bit Shift  mode=Shift Right Logical  N=7
  Constant1 : Constant  Value=51  OutDataTypeStr=uint8  SampleTime=-1
  Display : Display
  Multiport Switch1 : MultiPortSwitch  DataPortOrder=Zero-based contiguous  Inputs=29  DataPortForDefault=Additional data port  DiagnosticForDefault=Warning  zeroidx=on  SaturateOnIntegerOverflow=off  InputSameDT=off
  Scope : Scope
  Subtract : Sum  Inputs=+-  OutDataTypeStr=uint8  AccumDataTypeStr=uint8  RndMeth=Simplest  SaturateOnIntegerOverflow=on
  nibblepadding1 : Subsystem
  nibblepadding10 : Subsystem
  nibblepadding11 : Subsystem
  nibblepadding12 : Subsystem
  nibblepadding13 : Subsystem
  nibblepadding14 : Subsystem
  nibblepadding15 : Subsystem
  nibblepadding16 : Subsystem
  nibblepadding17 : Subsystem
  nibblepadding18 : Subsystem
  nibblepadding19 : Subsystem
  nibblepadding2 : Subsystem
  nibblepadding20 : Subsystem
  nibblepadding21 : Subsystem
  nibblepadding22 : Subsystem
  nibblepadding23 : Subsystem
  nibblepadding24 : Subsystem
  nibblepadding25 : Subsystem
  nibblepadding26 : Subsystem
  nibblepadding27 : Subsystem
  nibblepadding28 : Subsystem
  nibblepadding29 : Subsystem
  nibblepadding3 : Subsystem
  nibblepadding4 : Subsystem
  nibblepadding5 : Subsystem  Commented=on
  nibblepadding6 : Subsystem
  nibblepadding7 : Subsystem
  nibblepadding8 : Subsystem
  nibblepadding9 : Subsystem
  out : Outport
  wires:
  Multiport Switch1/1 -> out/1
  CTR/1 -> Subtract/2
  Bit Shift27/1 -> nibblepadding29/1(in)
  Bit Shift26/1 -> nibblepadding28/1(in)
  Bit Shift25/1 -> nibblepadding27/1(in)
  Bit Shift24/1 -> nibblepadding26/1(in)
  Bit Shift23/1 -> nibblepadding25/1(in)
  Bit Shift22/1 -> nibblepadding24/1(in)
  Bit Shift21/1 -> nibblepadding23/1(in)
  Bit Shift20/1 -> nibblepadding22/1(in)
  Bit Shift19/1 -> nibblepadding21/1(in)
  Bit Shift18/1 -> nibblepadding20/1(in)
  Bit Shift17/1 -> nibblepadding19/1(in)
  Bit Shift16/1 -> nibblepadding18/1(in)
  Bit Shift15/1 -> nibblepadding17/1(in)
  Bit Shift14/1 -> nibblepadding16/1(in)
  Bit Shift13/1 -> nibblepadding15/1(in)
  Bit Shift12/1 -> nibblepadding14/1(in)
  Bit Shift11/1 -> nibblepadding13/1(in)
  Bit Shift10/1 -> nibblepadding12/1(in)
  Bit Shift9/1 -> nibblepadding11/1(in)
  Bit Shift8/1 -> nibblepadding10/1(in)
  Bit Shift7/1 -> nibblepadding9/1(in)
  Bit Shift6/1 -> nibblepadding8/1(in)
  Bit Shift5/1 -> nibblepadding7/1(in)
  Bit Shift4/1 -> nibblepadding6/1(in)
  Bit Shift3/1 -> nibblepadding4/1(in)
  in/1 -> Multiport Switch1/31, nibblepadding1/1(in), nibblepadding2/1(in), nibblepadding3/1(in), Bit Shift26/1, Bit Shift27/1, Bit Shift25/1, Bit Shift24/1, Bit Shift23/1, Bit Shift22/1, Bit Shift21/1, Bit Shift20/1, Bit Shift19/1, Bit Shift18/1, Bit Shift17/1, Bit Shift16/1, Bit Shift15/1, Bit Shift14/1, Bit Shift13/1, Bit Shift12/1, Bit Shift11/1, Bit Shift10/1, Bit Shift9/1, Bit Shift8/1, Bit Shift7/1, Bit Shift6/1, Bit Shift5/1, Bit Shift4/1, Bit Shift3/1, Multiport Switch1/2
  in1/1 -> Add/2
  Constant1/1 -> Add/1
  Subtract/1 -> Display/1, Multiport Switch1/1, Scope/1
  Add/1 -> Subtract/1
  nibblepadding1/1(out) -> Multiport Switch1/3
  nibblepadding2/1(out) -> Multiport Switch1/4
  nibblepadding3/1(out) -> Multiport Switch1/5
  nibblepadding4/1(out) -> Multiport Switch1/6
  nibblepadding6/1(out) -> Multiport Switch1/7
  nibblepadding7/1(out) -> Multiport Switch1/8
  nibblepadding8/1(out) -> Multiport Switch1/9
  nibblepadding9/1(out) -> Multiport Switch1/10
  nibblepadding10/1(out) -> Multiport Switch1/11
  nibblepadding11/1(out) -> Multiport Switch1/12
  nibblepadding29/1(out) -> Multiport Switch1/30
  nibblepadding28/1(out) -> Multiport Switch1/29
  nibblepadding27/1(out) -> Multiport Switch1/28
  nibblepadding26/1(out) -> Multiport Switch1/27
  nibblepadding25/1(out) -> Multiport Switch1/26
  nibblepadding24/1(out) -> Multiport Switch1/25
  nibblepadding23/1(out) -> Multiport Switch1/24
  nibblepadding22/1(out) -> Multiport Switch1/23
  nibblepadding21/1(out) -> Multiport Switch1/22
  nibblepadding20/1(out) -> Multiport Switch1/21
  nibblepadding19/1(out) -> Multiport Switch1/20
  nibblepadding18/1(out) -> Multiport Switch1/19
  nibblepadding17/1(out) -> Multiport Switch1/18
  nibblepadding16/1(out) -> Multiport Switch1/17
  nibblepadding15/1(out) -> Multiport Switch1/16
  nibblepadding14/1(out) -> Multiport Switch1/15
  nibblepadding13/1(out) -> Multiport Switch1/14
  nibblepadding12/1(out) -> Multiport Switch1/13

== system UZ_EnDat_be4_adding_bidirectional_clk_shift/UZ_ENDAT_ABZ_ADDON/ManualSerialize1/padder1 ==
  in : Inport
  CTR : Inport  Port=2
  in1 : Inport  Port=3  OutDataTypeStr=int8
  Add : Sum  OutDataTypeStr=uint8  AccumDataTypeStr=uint8  RndMeth=Simplest
  Bit Shift10 : hdlsllib/Logic and Bit Operations/Bit Shift  mode=Shift Right Logical  N=8
  Bit Shift11 : hdlsllib/Logic and Bit Operations/Bit Shift  mode=Shift Right Logical  N=9
  Bit Shift12 : hdlsllib/Logic and Bit Operations/Bit Shift  mode=Shift Right Logical  N=10
  Bit Shift13 : hdlsllib/Logic and Bit Operations/Bit Shift  mode=Shift Right Logical  N=11
  Bit Shift14 : hdlsllib/Logic and Bit Operations/Bit Shift  mode=Shift Right Logical  N=12
  Bit Shift15 : hdlsllib/Logic and Bit Operations/Bit Shift  mode=Shift Right Logical  N=13
  Bit Shift16 : hdlsllib/Logic and Bit Operations/Bit Shift  mode=Shift Right Logical  N=14
  Bit Shift17 : hdlsllib/Logic and Bit Operations/Bit Shift  mode=Shift Right Logical  N=15
  Bit Shift18 : hdlsllib/Logic and Bit Operations/Bit Shift  mode=Shift Right Logical  N=16
  Bit Shift19 : hdlsllib/Logic and Bit Operations/Bit Shift  mode=Shift Right Logical  N=17
  Bit Shift20 : hdlsllib/Logic and Bit Operations/Bit Shift  mode=Shift Right Logical  N=18
  Bit Shift21 : hdlsllib/Logic and Bit Operations/Bit Shift  mode=Shift Right Logical  N=19
  Bit Shift22 : hdlsllib/Logic and Bit Operations/Bit Shift  mode=Shift Right Logical  N=20
  Bit Shift23 : hdlsllib/Logic and Bit Operations/Bit Shift  mode=Shift Right Logical  N=21
  Bit Shift24 : hdlsllib/Logic and Bit Operations/Bit Shift  mode=Shift Right Logical  N=22
  Bit Shift25 : hdlsllib/Logic and Bit Operations/Bit Shift  mode=Shift Right Logical  N=23
  Bit Shift26 : hdlsllib/Logic and Bit Operations/Bit Shift  mode=Shift Right Logical  N=24
  Bit Shift27 : hdlsllib/Logic and Bit Operations/Bit Shift  mode=Shift Right Logical  N=25
  Bit Shift3 : hdlsllib/Logic and Bit Operations/Bit Shift  mode=Shift Right Logical  N=1
  Bit Shift4 : hdlsllib/Logic and Bit Operations/Bit Shift  mode=Shift Right Logical  N=2
  Bit Shift5 : hdlsllib/Logic and Bit Operations/Bit Shift  mode=Shift Right Logical  N=3
  Bit Shift6 : hdlsllib/Logic and Bit Operations/Bit Shift  mode=Shift Right Logical  N=4
  Bit Shift7 : hdlsllib/Logic and Bit Operations/Bit Shift  mode=Shift Right Logical  N=5
  Bit Shift8 : hdlsllib/Logic and Bit Operations/Bit Shift  mode=Shift Right Logical  N=6
  Bit Shift9 : hdlsllib/Logic and Bit Operations/Bit Shift  mode=Shift Right Logical  N=7
  Constant1 : Constant  Value=51  OutDataTypeStr=uint8  SampleTime=-1
  Display : Display
  Multiport Switch1 : MultiPortSwitch  DataPortOrder=Zero-based contiguous  Inputs=29  DataPortForDefault=Additional data port  DiagnosticForDefault=Warning  zeroidx=on  SaturateOnIntegerOverflow=off  InputSameDT=off
  Scope : Scope
  Subtract : Sum  Inputs=+-  OutDataTypeStr=uint8  AccumDataTypeStr=uint8  RndMeth=Simplest  SaturateOnIntegerOverflow=on
  out : Outport
  wires:
  Multiport Switch1/1 -> out/1
  CTR/1 -> Subtract/2
  Bit Shift27/1 -> Multiport Switch1/30
  Bit Shift26/1 -> Multiport Switch1/29
  Bit Shift25/1 -> Multiport Switch1/28
  Bit Shift24/1 -> Multiport Switch1/27
  Bit Shift23/1 -> Multiport Switch1/26
  Bit Shift22/1 -> Multiport Switch1/25
  Bit Shift21/1 -> Multiport Switch1/24
  Bit Shift20/1 -> Multiport Switch1/23
  Bit Shift19/1 -> Multiport Switch1/22
  Bit Shift18/1 -> Multiport Switch1/21
  Bit Shift17/1 -> Multiport Switch1/20
  Bit Shift16/1 -> Multiport Switch1/19
  Bit Shift15/1 -> Multiport Switch1/18
  Bit Shift14/1 -> Multiport Switch1/17
  Bit Shift13/1 -> Multiport Switch1/16
  Bit Shift12/1 -> Multiport Switch1/15
  Bit Shift11/1 -> Multiport Switch1/14
  Bit Shift10/1 -> Multiport Switch1/13
  Bit Shift9/1 -> Multiport Switch1/12
  Bit Shift8/1 -> Multiport Switch1/11
  Bit Shift7/1 -> Multiport Switch1/10
  Bit Shift6/1 -> Multiport Switch1/9
  Bit Shift5/1 -> Multiport Switch1/8
  Bit Shift4/1 -> Multiport Switch1/7
  Bit Shift3/1 -> Multiport Switch1/6
  in/1 -> Multiport Switch1/31, Multiport Switch1/3, Multiport Switch1/4, Multiport Switch1/5, Bit Shift26/1, Bit Shift27/1, Bit Shift25/1, Bit Shift24/1, Bit Shift23/1, Bit Shift22/1, Bit Shift21/1, Bit Shift20/1, Bit Shift19/1, Bit Shift18/1, Bit Shift17/1, Bit Shift16/1, Bit Shift15/1, Bit Shift14/1, Bit Shift13/1, Bit Shift12/1, Bit Shift11/1, Bit Shift10/1, Bit Shift9/1, Bit Shift8/1, Bit Shift7/1, Bit Shift6/1, Bit Shift5/1, Bit Shift4/1, Bit Shift3/1, Multiport Switch1/2
  in1/1 -> Add/2
  Constant1/1 -> Add/1
  Subtract/1 -> Display/1, Multiport Switch1/1, Scope/1
  Add/1 -> Subtract/1

== system UZ_EnDat_be4_adding_bidirectional_clk_shift/UZ_ENDAT_ABZ_ADDON/ManualSerialize1/padding2 ==
  in : Inport
  Bit Shift2 : hdlsllib/Logic and Bit Operations/Bit Shift  mode=Shift Right Logical  N=1
  Bit Slice2 : hdlsllib/Logic and Bit Operations/Bit Slice  lidx=0  ridx=0
  Data Type Conversion2 : DataTypeConversion  OutDataTypeStr=boolean  RndMeth=Nearest  SaturateOnIntegerOverflow=off
  Switch2 : Switch  Criteria=u2 > Threshold  SaturateOnIntegerOverflow=off  InputSameDT=off
  out : Outport
  wires:
  in/1 -> Bit Shift2/1, Switch2/1, Bit Slice2/1
  Bit Shift2/1 -> Switch2/3
  Data Type Conversion2/1 -> Switch2/2
  Bit Slice2/1 -> Data Type Conversion2/1
  Switch2/1 -> out/1

== system UZ_EnDat_be4_adding_bidirectional_clk_shift/UZ_ENDAT_ABZ_ADDON/ManualSerialize1/padding5 ==
  in : Inport
  Bit Shift1 : hdlsllib/Logic and Bit Operations/Bit Shift  mode=Shift Right Logical  N=2
  Bit Shift2 : hdlsllib/Logic and Bit Operations/Bit Shift  mode=Shift Right Logical  N=1
  Bit Shift3 : hdlsllib/Logic and Bit Operations/Bit Shift  mode=Shift Right Logical  N=3
  Bit Slice1 : hdlsllib/Logic and Bit Operations/Bit Slice  lidx=0  ridx=0
  Bit Slice3 : hdlsllib/Logic and Bit Operations/Bit Slice  lidx=1  ridx=0
  Bit Slice4 : hdlsllib/Logic and Bit Operations/Bit Slice  lidx=2  ridx=0
  Compare To Zero : hdlsllib/Logic and Bit Operations/Compare To Zero  relop=<=  OutDataTypeStr=boolean
  Compare To Zero1 : hdlsllib/Logic and Bit Operations/Compare To Zero  relop=<=  OutDataTypeStr=boolean
  Compare To Zero2 : hdlsllib/Logic and Bit Operations/Compare To Zero  relop=<=  OutDataTypeStr=boolean
  Logical Operator : Logic  Inputs=3  AllPortsSameDT=off  OutDataTypeStr=boolean
  Logical Operator1 : Logic  Operator=NOT  Inputs=3  AllPortsSameDT=off  OutDataTypeStr=boolean
  Logical Operator2 : Logic  Operator=NOT  Inputs=3  AllPortsSameDT=off  OutDataTypeStr=boolean
  Logical Operator3 : Logic  Inputs=3  AllPortsSameDT=off  OutDataTypeStr=boolean
  Logical Operator4 : Logic  Inputs=3  AllPortsSameDT=off  OutDataTypeStr=boolean
  Switch1 : Switch  Criteria=u2 > Threshold  SaturateOnIntegerOverflow=off  InputSameDT=off
  Switch2 : Switch  Criteria=u2 > Threshold  SaturateOnIntegerOverflow=off  InputSameDT=off
  Switch3 : Switch  Criteria=u2 > Threshold  SaturateOnIntegerOverflow=off  InputSameDT=off
  out : Outport
  wires:
  in/1 -> Bit Slice4/1, Bit Slice3/1, Bit Slice1/1, Switch2/3, Bit Shift2/1
  Bit Shift2/1 -> Switch2/1
  Switch2/1 -> Switch1/3, Bit Shift1/1
  Bit Slice3/1 -> Compare To Zero/1
  Bit Slice4/1 -> Compare To Zero1/1
  Bit Slice1/1 -> Compare To Zero2/1
  Compare To Zero2/1 -> Logical Operator4/2, Logical Operator3/1, Logical Operator/1
  Compare To Zero/1 -> Logical Operator4/1, Logical Operator3/2, Logical Operator1/1
  Logical Operator1/1 -> Logical Operator/3
  Compare To Zero1/1 -> Logical Operator4/3, Logical Operator2/1
  Logical Operator2/1 -> Logical Operator/2, Logical Operator3/3
  Logical Operator/1 -> Switch2/2
  Bit Shift1/1 -> Switch1/1
  Logical Operator3/1 -> Switch1/2
  Switch1/1 -> Switch3/3, Bit Shift3/1
  Bit Shift3/1 -> Switch3/1
  Logical Operator4/1 -> Switch3/2
  Switch3/1 -> out/1

== system UZ_EnDat_be4_adding_bidirectional_clk_shift/UZ_ENDAT_ABZ_ADDON/ManualSerialize1/prolonger ==
  in : Inport
  Delay4 : Delay  DelayLength=1
  Logical Operator5 : Logic  Operator=OR  AllPortsSameDT=off  OutDataTypeStr=boolean
  out : Outport
  wires:
  Logical Operator5/1 -> out/1
  in/1 -> Delay4/1, Logical Operator5/1
  Delay4/1 -> Logical Operator5/2

== system UZ_EnDat_be4_adding_bidirectional_clk_shift/UZ_ENDAT_ABZ_ADDON/responseslicer5/ENDAT23BITREVERSER ==
  in : Inport
  32BITREVERSE : Subsystem
  Bit Shift : hdlsllib/Logic and Bit Operations/Bit Shift  mode=Shift Right Logical  N=8
  Data Type Conversion : DataTypeConversion  OutDataTypeStr=uint32  RndMeth=Nearest  SaturateOnIntegerOverflow=off
  out : Outport
  wires:
  Bit Shift/1 -> out/1
  in/1 -> Data Type Conversion/1
  32BITREVERSE/1(out) -> Bit Shift/1
  Data Type Conversion/1 -> 32BITREVERSE/1(in)

== system UZ_EnDat_be4_adding_bidirectional_clk_shift/UZ_ENDAT/CLKGEN/CLKDIV1/Triggered Subsystem ==
  IN : Inport
  Trigger : TriggerPort  VariantControl=(inherit)  OutputDataType=int8  InitialTriggerSignalState=positive
  OUT : Outport  InitialOutput=0
  wires:
  IN/1 -> OUT/1

== system UZ_EnDat_be4_adding_bidirectional_clk_shift/UZ_ENDAT/CLKGEN/CLKDIV3/Triggered Subsystem ==
  IN : Inport
  Trigger : TriggerPort  VariantControl=(inherit)  OutputDataType=int8  InitialTriggerSignalState=positive
  OUT : Outport  InitialOutput=0
  wires:
  IN/1 -> OUT/1

== system UZ_EnDat_be4_adding_bidirectional_clk_shift/UZ_ENDAT/CLKGEN/CLKDIV4/Triggered Subsystem ==
  IN : Inport
  Trigger : TriggerPort  VariantControl=(inherit)  OutputDataType=int8  InitialTriggerSignalState=positive
  OUT : Outport  InitialOutput=0
  wires:
  IN/1 -> OUT/1

== system UZ_EnDat_be4_adding_bidirectional_clk_shift/UZ_ENDAT/CLKGEN/CLKDIV5/Triggered Subsystem ==
  IN : Inport
  Trigger : TriggerPort  VariantControl=(inherit)  OutputDataType=int8  InitialTriggerSignalState=positive
  OUT : Outport  InitialOutput=0
  wires:
  IN/1 -> OUT/1

== system UZ_EnDat_be4_adding_bidirectional_clk_shift/UZ_ENDAT/CLKGEN/CLKDIV6/Triggered Subsystem ==
  IN : Inport
  Trigger : TriggerPort  VariantControl=(inherit)  OutputDataType=int8  InitialTriggerSignalState=positive
  OUT : Outport  InitialOutput=0
  wires:
  IN/1 -> OUT/1

== system UZ_EnDat_be4_adding_bidirectional_clk_shift/UZ_ENDAT/CLKGEN/CLKDIV7/Triggered Subsystem ==
  IN : Inport
  Trigger : TriggerPort  VariantControl=(inherit)  OutputDataType=int8  InitialTriggerSignalState=positive
  OUT : Outport  InitialOutput=0
  wires:
  IN/1 -> OUT/1

== system UZ_EnDat_be4_adding_bidirectional_clk_shift/UZ_ENDAT/CLKGEN/CLKDIV8/Triggered Subsystem ==
  IN : Inport
  Trigger : TriggerPort  VariantControl=(inherit)  OutputDataType=int8  InitialTriggerSignalState=positive
  OUT : Outport  InitialOutput=0
  wires:
  IN/1 -> OUT/1

== system UZ_EnDat_be4_adding_bidirectional_clk_shift/UZ_ENDAT/CLKGEN/CLKDIV9/Triggered Subsystem ==
  IN : Inport
  Trigger : TriggerPort  VariantControl=(inherit)  OutputDataType=int8  InitialTriggerSignalState=positive
  OUT : Outport  InitialOutput=0
  wires:
  IN/1 -> OUT/1
